simulink model "cdip_pcont_sim"  (R2013a)
settings: Solver=ode4  StartTime=0.0  StopTime=4  FixedStep=0.001  RelTol=1e-3
values from neighbouring files (symbols this model uses):
  ac = 2*zeta*omega_n    [p1c321_cdip_id_cart.m]    (also in p1c322_cdip_id_least_square.m = p1(1))
  bc = omega_n^2/kP    [p1c321_cdip_id_cart.m]    (also in p1c322_cdip_id_least_square.m = p1(2))
  dtheta_0 = 0    [p1c322_cdip_id_least_square.m]    (also in p1c34_cdip_plot_pcont.m)
  dz_0 = 0    [p1c322_cdip_id_least_square.m]    (also in p1c34_cdip_plot_pcont.m)
  g = 9.81e+000    (= 9.81)    [p1c321_cdip_id_pend.m]    (also in p1c322_cdip_id_least_square.m; p1c322_cdip_plot_MN.m; p1c332_adip_id_least_square.m; p1c332_adip_id_pend.m)
  Jp = mp*g*lp/omega_n^2 - mp*lp^2    [p1c321_cdip_id_pend.m]    (also in p1c322_cdip_id_least_square.m = p2(1))
  lp = 2.30e-001    (= 0.23)    [p1c321_cdip_id_pend.m]    (also in p1c322_cdip_id_least_square.m; p1c322_cdip_plot_MN.m)
  mp = 1.07e-001    (= 0.107)    [p1c321_cdip_id_pend.m]    (also in p1c322_cdip_id_least_square.m; p1c322_cdip_plot_MN.m)
  mup = 2*zeta*omega_n*(Jp + mp*lp^2)    [p1c321_cdip_id_pend.m]    (also in p1c322_cdip_id_least_square.m = p2(2))
  theta_0 = pi    (= 3.14159265359)    [p1c322_cdip_id_least_square.m]    (also in p1c34_cdip_plot_pcont.m)
  z_0 = 0    [p1c322_cdip_id_least_square.m]    (also in p1c34_cdip_plot_pcont.m)
settings Model: ExtModeTrigDuration=5000  Creator=student  LastModifiedBy=kawata
settings SolverCC: PositivePriorityOrder=on
settings DataIOCC: SignalLoggingSaveFormat=ModelDataLogs
settings OptimizationCC: ExpressionDepthLimit=2147483647
settings DebuggingCC: FcnCallInpInsideContextMsg=UseLocalSettings  FrameProcessingCompatibilityMsg=error
settings GRTTargetCC: CodeReplacementLibrary=C89/C90 (ANSI)  CombineOutputUpdateFcns=off  GRTInterface=on

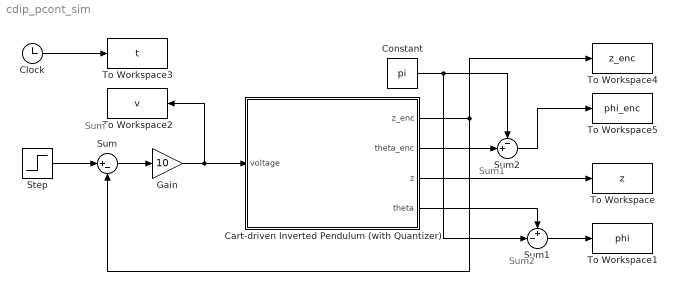
== system cdip_pcont_sim ==
  note: Sum
  note: Sum1
  note: Sum2
  Cart-driven Inverted Pendulum (with Quantizer) : Subsystem
      mask Display: image(imread('cdip_photo.jpg'),'center')
  Clock : Clock
  Constant : Constant  Value=pi
  Gain : Gain  Gain=10  SaturateOnIntegerOverflow=on  OutDataTypeStr=Inherit: Same as input  ParamDataTypeStr=Inherit: Same as input
  Step : Step  Time=0  After=0.2  SampleTime=0
  Sum : Sum  Inputs=|+-  SaturateOnIntegerOverflow=on  InputSameDT=on  OutDataTypeStr=Inherit: Same as first input
  Sum1 : Sum  Inputs=+-|  SaturateOnIntegerOverflow=on  InputSameDT=on  OutDataTypeStr=Inherit: Same as first input
  Sum2 : Sum  Inputs=-+|  SaturateOnIntegerOverflow=on  InputSameDT=on  OutDataTypeStr=Inherit: Same as first input
  To Workspace : ToWorkspace  VariableName=z  SampleTime=-1
  To Workspace1 : ToWorkspace  VariableName=phi  SampleTime=-1
  To Workspace2 : ToWorkspace  VariableName=v  SampleTime=-1
  To Workspace3 : ToWorkspace  VariableName=t  SampleTime=-1
  To Workspace4 : ToWorkspace  VariableName=z_enc  SampleTime=-1
  To Workspace5 : ToWorkspace  VariableName=phi_enc  SampleTime=-1
  wires:
  Step/1 -> Sum/1
  Sum/1 -> Gain/1
  Gain/1 -> Cart-driven Inverted Pendulum (with Quantizer)/1(voltage), To Workspace2/1
  Clock/1 -> To Workspace3/1
  Sum1/1 -> To Workspace1/1
  Cart-driven Inverted Pendulum (with Quantizer)/3(z) -> To Workspace/1
  Cart-driven Inverted Pendulum (with Quantizer)/1(z_enc) -> To Workspace4/1, Sum/2
  Cart-driven Inverted Pendulum (with Quantizer)/4(theta) -> Sum1/1
  Constant/1 -> Sum2/1, Sum1/2
  Cart-driven Inverted Pendulum (with Quantizer)/2(theta_enc) -> Sum2/2
  Sum2/1 -> To Workspace5/1

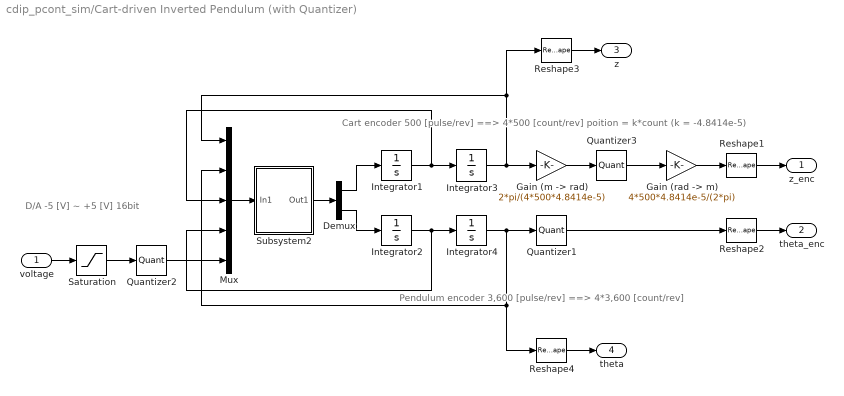
== system cdip_pcont_sim/Cart-driven Inverted Pendulum (with Quantizer) ==
  note: Cart encoder
      |   500 [pulse/rev]  ==> 4*500 [count/rev]
      |   poition = k*count  (k = -4.8414e-5)
  note: D/A
      |   -5 [V] ~ +5 [V]
      |  16bit
  note: Pendulum encoder
      |   3,600 [pulse/rev]  ==> 4*3,600 [count/rev]
  voltage : Inport
  Demux : Demux  Outputs=2
  "Gain (m -> rad)" : Gain  Gain=2*pi/(4*500*4.8414e-5)  SaturateOnIntegerOverflow=on  OutDataTypeStr=Inherit: Same as input  ParamDataTypeStr=Inherit: Same as input
  "Gain (rad -> m)" : Gain  Gain=4*500*4.8414e-5/(2*pi)  SaturateOnIntegerOverflow=on  OutDataTypeStr=Inherit: Same as input  ParamDataTypeStr=Inherit: Same as input
  Integrator1 : Integrator  InitialCondition=dz_0
  Integrator2 : Integrator  InitialCondition=dtheta_0
  Integrator3 : Integrator  InitialCondition=z_0
  Integrator4 : Integrator  InitialCondition=theta_0
  Mux : Mux  Inputs=5
  Quantizer1 : Quantizer  QuantizationInterval=2*pi/(4*3600)
  Quantizer2 : Quantizer  QuantizationInterval=10/2^(16)
  Quantizer3 : Quantizer  QuantizationInterval=2*pi/(4*500)
  Reshape{1..4} (4 alike) : Reshape
  Saturation : Saturate  UpperLimit=5  LowerLimit=-5
  Subsystem2 : Subsystem
  z_enc : Outport
  theta_enc : Outport  Port=2
  z : Outport  Port=3
  theta : Outport  Port=4
  wires:
  Reshape4/1 -> theta/1
  Reshape3/1 -> z/1
  Saturation/1 -> Quantizer2/1
  Quantizer2/1 -> Mux/5
  Quantizer1/1 -> Reshape2/1
  Subsystem2/1(Out1) -> Demux/1
  Mux/1 -> Subsystem2/1(In1)
  Demux/1 -> Integrator1/1
  Demux/2 -> Integrator2/1
  Integrator1/1 -> Mux/3, Integrator3/1
  Integrator2/1 -> Mux/4, Integrator4/1
  Integrator3/1 -> Reshape3/1, Mux/1, "Gain (m -> rad)"/1
  Integrator4/1 -> Reshape4/1, Mux/2, Quantizer1/1
  voltage/1 -> Saturation/1
  "Gain (m -> rad)"/1 -> Quantizer3/1
  Quantizer3/1 -> "Gain (rad -> m)"/1
  "Gain (rad -> m)"/1 -> Reshape1/1
  Reshape1/1 -> z_enc/1
  Reshape2/1 -> theta_enc/1

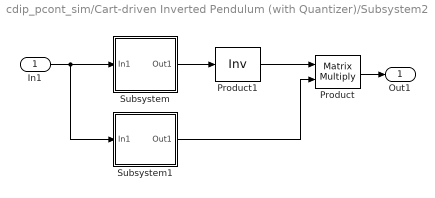
== system cdip_pcont_sim/Cart-driven Inverted Pendulum (with Quantizer)/Subsystem2 ==
  In1 : Inport
  Product : Product  Multiplication=Matrix(*)  SaturateOnIntegerOverflow=on  InputSameDT=on  OutDataTypeStr=Inherit: Same as first input
  Product1 : Product  Inputs=/  Multiplication=Matrix(*)  SaturateOnIntegerOverflow=on  InputSameDT=on  OutDataTypeStr=Inherit: Same as first input
  Subsystem : Subsystem
  Subsystem1 : Subsystem
  Out1 : Outport
  wires:
  Subsystem/1(Out1) -> Product1/1
  Product1/1 -> Product/1
  Subsystem1/1(Out1) -> Product/2
  In1/1 -> Subsystem/1(In1), Subsystem1/1(In1)
  Product/1 -> Out1/1

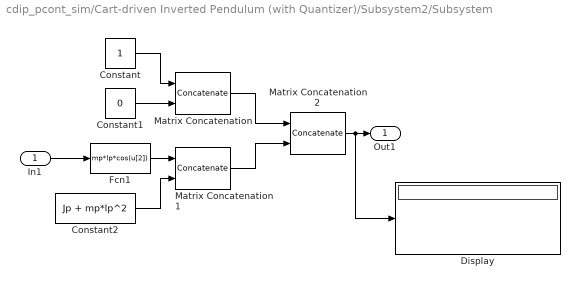
== system cdip_pcont_sim/Cart-driven Inverted Pendulum (with Quantizer)/Subsystem2/Subsystem ==
  In1 : Inport
  Constant : Constant
  Constant1 : Constant  Value=0
  Constant2 : Constant  Value=Jp + mp*lp^2
  Display : Display
  Fcn1 : Fcn  Expr=mp*lp*cos(u[2])
  Matrix Concatenation : Concatenate  Mode=Multidimensional array  ConcatenateDimension=2
  Matrix Concatenation1 : Concatenate  Mode=Multidimensional array  ConcatenateDimension=2
  Matrix Concatenation2 : Concatenate  Mode=Multidimensional array
  Out1 : Outport
  wires:
  Constant2/1 -> Matrix Concatenation1/2
  Fcn1/1 -> Matrix Concatenation1/1
  In1/1 -> Fcn1/1
  Matrix Concatenation/1 -> Matrix Concatenation2/1
  Matrix Concatenation1/1 -> Matrix Concatenation2/2
  Matrix Concatenation2/1 -> Display/1, Out1/1
  Constant/1 -> Matrix Concatenation/1
  Constant1/1 -> Matrix Concatenation/2

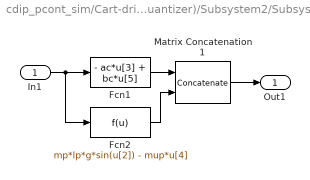
== system cdip_pcont_sim/Cart-driven Inverted Pendulum (with Quantizer)/Subsystem2/Subsystem1 ==
  In1 : Inport
  Fcn1 : Fcn  Expr=- ac*u[3] + bc*u[5]
  Fcn2 : Fcn  Expr=mp*lp*g*sin(u[2]) - mup*u[4]
  Matrix Concatenation1 : Concatenate  Mode=Multidimensional array
  Out1 : Outport
  wires:
  Fcn2/1 -> Matrix Concatenation1/2
  Fcn1/1 -> Matrix Concatenation1/1
  In1/1 -> Fcn2/1, Fcn1/1
  Matrix Concatenation1/1 -> Out1/1
